simulink model "CSRT_NL"  (R2020b)
settings: Solver=FixedStepAuto  StartTime=0.0  StopTime=15  FixedStep=0.01  RelTol=1e-3
values from neighbouring files (symbols this model uses):
  Cafs = 10    [Exp2_CSRT.m]
  Cas = 8.564    [Exp2_CSRT.m]
  Fs = 1    [Exp2_CSRT.m]
  Tfs = 298    [Exp2_CSRT.m]
  Tjs = 298    [Exp2_CSRT.m]
  Ts = 311.2    [Exp2_CSRT.m]
settings Model: Creator=franc  LastModifiedBy=franc

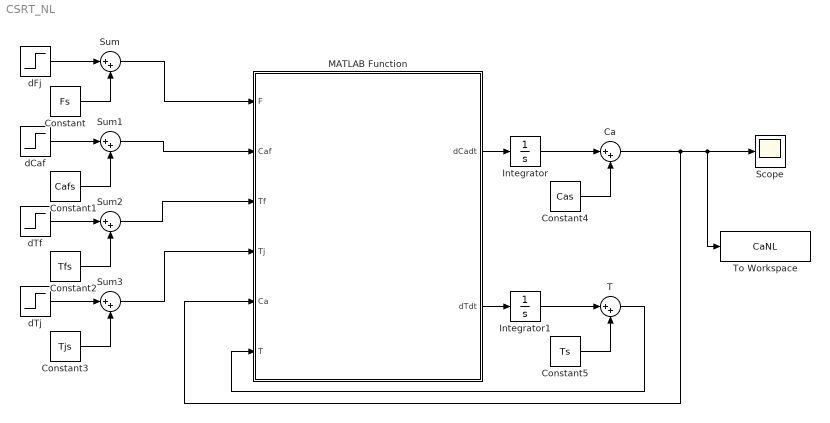
== system CSRT_NL ==
  "              Ca" : Sum  Inputs=|++
  "            T" : Sum  Inputs=|++
  Constant : Constant  Value=Fs
  Constant1 : Constant  Value=Cafs
  Constant2 : Constant  Value=Tfs
  Constant3 : Constant  Value=Tjs
  Constant4 : Constant  Value=Cas
  Constant5 : Constant  Value=Ts
  Integrator : Integrator
  Integrator1 : Integrator
  MATLAB Function : MATLAB Function  TreatAsAtomicUnit=on
  Scope : Scope
  Sum{,1..3} (4 alike) : Sum  Inputs=|++
  To Workspace : ToWorkspace  VariableName=CaNL  SaveFormat=Timeseries  SampleTime=-1
  dCaf : Step  Time=0  After=0  SampleTime=0
  dFj : Step  Time=0  After=0.01  SampleTime=0
  dTf : Step  Time=0  After=0  SampleTime=0
  dTj : Step  Time=0  After=0  SampleTime=0
  wires:
  dFj/1 -> Sum/1
  Constant/1 -> Sum/2
  Sum/1 -> MATLAB Function/1(F)
  Constant1/1 -> Sum1/2
  dCaf/1 -> Sum1/1
  Sum1/1 -> MATLAB Function/2(Caf)
  Constant2/1 -> Sum2/2
  dTf/1 -> Sum2/1
  Sum2/1 -> MATLAB Function/3(Tf)
  dTj/1 -> Sum3/1
  Constant3/1 -> Sum3/2
  Sum3/1 -> MATLAB Function/4(Tj)
  Integrator/1 -> "              Ca"/1
  MATLAB Function/1(dCadt) -> Integrator/1
  Constant4/1 -> "              Ca"/2
  "              Ca"/1 -> MATLAB Function/5(Ca), To Workspace/1, Scope/1
  MATLAB Function/2(dTdt) -> Integrator1/1
  Integrator1/1 -> "            T"/1
  Constant5/1 -> "            T"/2
  "            T"/1 -> MATLAB Function/6(T)

== matlab function CSRT_NL/MATLAB Function ==
  data: F input; dCadt output; dTdt output; Caf input; Tf input; Tj input; Ca input; T input
function [dCadt, dTdt] = fcn(F, Caf, Tf, Tj, Ca, T)
% Definição dos parâmetros do reator
V     = 1;         % Volume do reator (m^3)
dE    = 11843;     % Energia de ativação (J/mol)
rhocp = 500;       % Densidade*Capacidade térmica (J/(K*m^3))
R     = 1.987;     % Constante de gás ideal (L/(mol*K))
UA    = 150;       % Coef. geral transf. calor*área para troca de calor (J/(Kh))
k0    = 9703*3600; % Fator pré-exponencial (h^-1)
dH    = -5960;     % Calor de reação (J/mol)

r = k0*exp(-dE/(R*T))*Ca;

dCadt = (F/V)*(Caf - Ca) - r;
dTdt  = (F/V)*(Tf - T) + (-dH/rhocp)*r - (UA/(V*rhocp))*(T - Tj);
